simulink model "b4Vor_block_diagram"  (Simulink 8.0)
settings: Solver=ode45  StartTime=0.0  StopTime=10.0  RelTol=1e-3
values from neighbouring files (symbols this model uses):
  delay = 0.007    [codeB.m]
  g = 1    [canal_afferent_step_response.m]    (also in codeA.m; codeB.m = -5)
  T = 0.015    [canal_afferent_step_response.m]    (also in codeA.m; codeB.m)
  T2 = 0.003    [canal_afferent_step_response.m]    (also in codeA.m; codeB.m)
  Tc = 5.7    [codeB.m]
  Te1 = 20    [codeB.m]
  Te2 = 0.016    [codeB.m]
  Ts = 1/fs    (= 0.001)    [canal_afferent_step_response.m]    (also in codeA.m; codeB.m)
  Tvor = 20    [codeB.m]
settings Model: Creator=wang0_000  LastModifiedBy=wang0_000
settings DataIOCC: SignalLoggingSaveFormat=ModelDataLogs
settings OptimizationCC: InitFltsAndDblsToZero=on
settings DebuggingCC: SaveWithParameterizedLinksMsg=none  SignalResolutionControl=TryResolveAllWithWarning  MultiTaskDSMMsg=warning  MultiTaskCondExecSysMsg=none  FcnCallInpInsideContextMsg=UseLocalSettings  StrictBusMsg=None
settings RTWCC: IncludeERTFirstTime=on
settings GRTTargetCC: TargetFcnLib=ansi_tfl_tmw.mat  CombineOutputUpdateFcns=off  GRTInterface=on

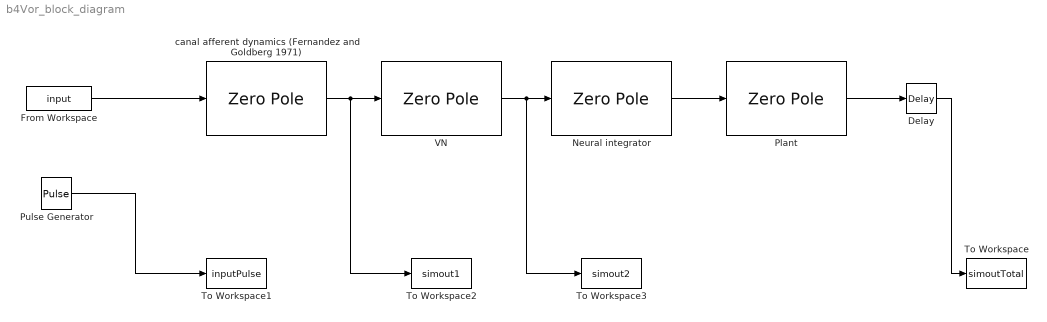
== system b4Vor_block_diagram ==
  Delay : TransportDelay  DelayTime=delay
  From Workspace : FromWorkspace  VariableName=input  SampleTime=0
  Neural integrator : ZeroPole  Zeros=[-1/Te1]  Poles=[0]  Gain=[Te1]
  Plant : ZeroPole  Zeros=[0]  Poles=[-1/Te1 -1/Te2]  Gain=[1/(Te1*Te2)]
  Pulse Generator : DiscretePulseGenerator  PulseType=Time based  Period=100  PulseWidth=50  PhaseDelay=10
  To Workspace : ToWorkspace  VariableName=simoutTotal  SampleTime=Ts
  To Workspace1 : ToWorkspace  VariableName=inputPulse  SampleTime=Ts
  To Workspace2 : ToWorkspace  VariableName=simout1  SampleTime=Ts
  To Workspace3 : ToWorkspace  VariableName=simout2  SampleTime=Ts
  VN : ZeroPole  Zeros=[-1/Tc]  Poles=[-1/Tvor ]  Gain=[-g]
  canal afferent dynamics (Fernandez and Goldberg 1971) : ZeroPole  Zeros=[ 0 -1/T]  Poles=[-1/Tc -1/T2]  Gain=[T/(Tc*T2)]
  wires:
  canal afferent dynamics (Fernandez and Goldberg 1971)/1 -> To Workspace2/1, VN/1
  Plant/1 -> Delay/1
  Delay/1 -> To Workspace/1
  VN/1 -> To Workspace3/1, Neural integrator/1
  Neural integrator/1 -> Plant/1
  Pulse Generator/1 -> To Workspace1/1
  From Workspace/1 -> canal afferent dynamics (Fernandez and Goldberg 1971)/1
